simulink model "PthSet"  (R2018a)
settings: configuration reference "cs_ert" (kept outside this file)
settings Model: DataDictionary=PthSet.sldd  Creator=zhoutinglin  LastModifiedBy=zhoutinglin

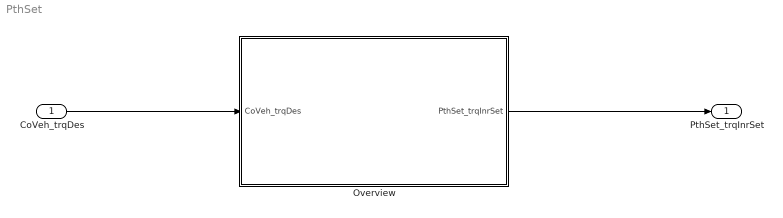
== system PthSet ==
  CoVeh_trqDes : Inport
  Overview : Subsystem
  PthSet_trqInrSet : Outport
  wires:
  CoVeh_trqDes/1 -> Overview/1(CoVeh_trqDes)
  Overview/1(PthSet_trqInrSet) -> PthSet_trqInrSet/1

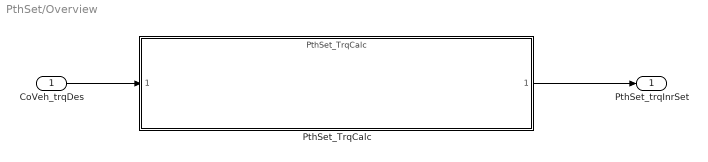
== system PthSet/Overview ==
  CoVeh_trqDes : Inport
  PthSet_TrqCalc : ModelReference  ModelNameDialog=PthSet_TrqCalc  SimulationMode=Normal  ModelReferenceVersion=1.55
  PthSet_trqInrSet : Outport
  wires:
  CoVeh_trqDes/1 -> PthSet_TrqCalc/1
  PthSet_TrqCalc/1 -> PthSet_trqInrSet/1
